simulink model "ex1_sim"  (R2022b)
settings: Solver=VariableStepAuto  StartTime=0.0  StopTime=20  RelTol=1e-3
undefined symbols (not defined in the file): den_tf, kp, Kw, num_tf, Td, Ti, Tl
libraries: simulink x1
settings Model: Creator=david  LastModifiedBy=david

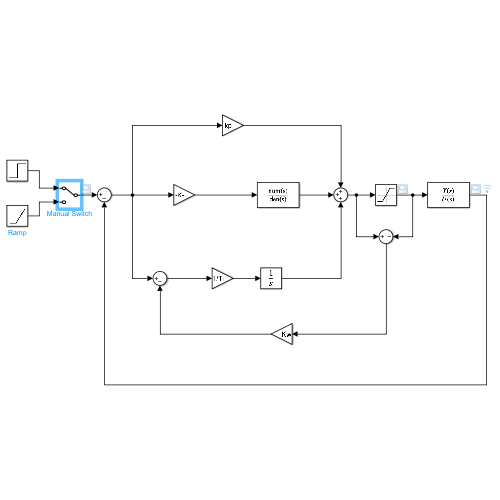
[thumbnail: Simulink's stored preview of the top-level diagram]
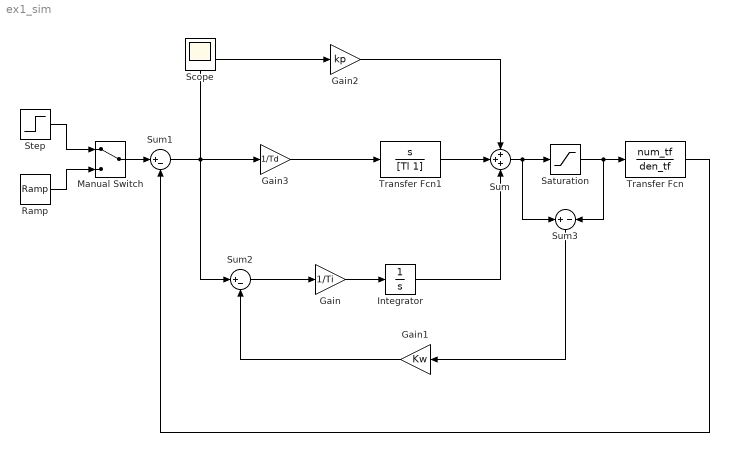
== system ex1_sim ==
  Gain : Gain  Gain=1/Ti
  Gain1 : Gain  Gain=Kw
  Gain2 : Gain  Gain=kp
  Gain3 : Gain  Gain=1/Td
  Integrator : Integrator
  Manual Switch : ManualSwitch
  Ramp : simulink/Sources/Ramp  slope=1  start=0  InitialOutput=0
  Saturation : Saturate  UpperLimit=10  LowerLimit=-10
  Step : Step  SampleTime=0
  Sum : Sum  Inputs=+++
  Sum1 : Sum  Inputs=|+-
  Sum2 : Sum  Inputs=|+-
  Sum3 : Sum  Inputs=+|-
  Transfer Fcn : TransferFcn  Numerator=num_tf  Denominator=den_tf
  Transfer Fcn1 : TransferFcn  Numerator=[1, 0]  Denominator=[Tl 1]
  Scope : Scope
  wires:
  Sum/1 -> Sum3/1, Saturation/1
  Saturation/1 -> Sum3/2, Transfer Fcn/1
  Gain/1 -> Integrator/1
  Integrator/1 -> Sum/3
  Step/1 -> Manual Switch/1
  Ramp/1 -> Manual Switch/2
  Manual Switch/1 -> Sum1/1
  Sum3/1 -> Gain1/1
  Gain1/1 -> Sum2/2
  Sum2/1 -> Gain/1
  Sum1/1 -> Gain3/1, Sum2/1, Gain2/1
  Transfer Fcn/1 -> Sum1/2
  Gain2/1 -> Sum/1
  Gain3/1 -> Transfer Fcn1/1
  Transfer Fcn1/1 -> Sum/2
